simulink model "UDP1"  (R2024b)
settings: Solver=FixedStepAuto  StartTime=0.0  StopTime=inf  FixedStep=0.01  RelTol=1e-3
undefined symbols (not defined in the file or in its folder): f
libraries: etargetslib x1, instrumentlib x1
settings Model: Creator=hamza  LastModifiedBy=hamza

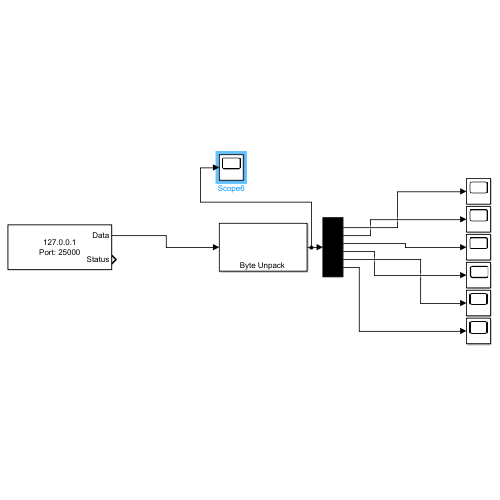
[thumbnail: Simulink's stored preview of the top-level diagram]
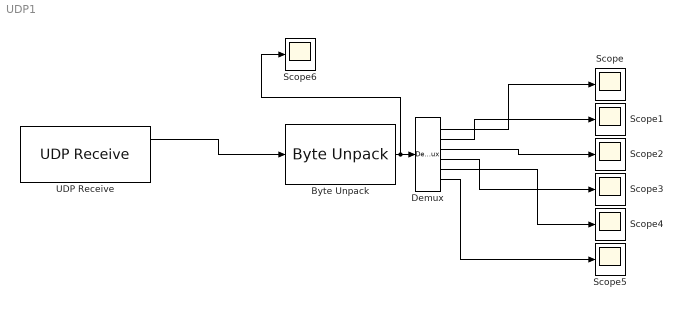
== system UDP1 ==
  Byte Unpack : etargetslib/Byte Unpack  dimensions={[6]}  datatypes={'single'}  byteAlign=4
      settings: LibrarySourceBlock=embeddedtargetslib/Host Communication/Byte Unpack
  Demux : Demux  Outputs=6
  Scope{,1..6} (7 alike) : Scope
  UDP Receive : instrumentlib/UDP Receive  LocalAddress=127.0.0.1  LocalPort=25000  EnablePortSharing=off  Host=localhost  Port=9090  GetLatestData=off  DataSize=[ 24, 1 ]  DataType=uint8  ASCIIFormatting=%f,  Terminator=LF  CustomTerminator=10  ByteOrder=big-endian  EnableBlockingMode=off  Timeout=1  SampleTime=0.01  SimulateUsing=Interpreted execution
  wires:
  UDP Receive/1 -> Byte Unpack/1
  Byte Unpack/1 -> Scope6/1, Demux/1
  Demux/1 -> Scope/1
  Demux/2 -> Scope1/1
  Demux/3 -> Scope2/1
  Demux/4 -> Scope3/1
  Demux/5 -> Scope4/1
  Demux/6 -> Scope5/1
